simulink model "TST_EnumTypes"  (Simulink 7.4)
settings: Solver=FixedStepDiscrete  StartTime=0.0  StopTime=10.0  FixedStep=0.02  RelTol=1e-3
undefined symbols (not defined in the file): DIL_VmmGsFcsCommandsMessage_LatApModeCmd, DIL_VmmGsFcsCommandsMessage_LongApModeCmd
settings Model: Creator=kharthforeign  LastModifiedBy=kharthforeign  BufferReuse=off
settings DataIOCC: SaveOutput=off  SignalLogging=off  SaveTime=off
settings OptimizationCC: BlockReduction=off  ConditionallyExecuteInputs=off  OptimizeBlockIOStorage=off  BufferReuse=off  ExpressionFolding=off  LocalBlockOutputs=off  InitFltsAndDblsToZero=on

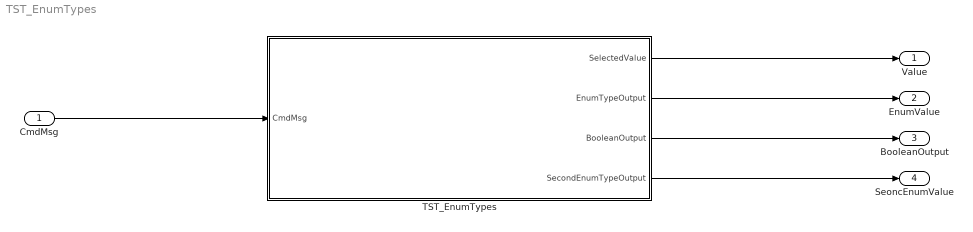
== system TST_EnumTypes ==
  CmdMsg : Inport  UseBusObject=on  OutDataType=fixdt(1, 16)  OutScaling=2^0  BusOutputAsStruct=on
      settings: BusObject=DIL_VmmGsFcsCommandsMessage_Data
  TST_EnumTypes : Subsystem  TreatAsAtomicUnit=on
  Value : Outport  PortDimensions=1  DataType=double  OutDataType=fixdt(1, 16)  OutScaling=2^0  OutDataTypeStr=double
  EnumValue : Outport  Port=2  PortDimensions=1  DataType=Specify via dialog  OutDataType=Enum: DIL_VmmGsFcsCommandsMessage_LongApModeCmd  OutDataTypeStr=Enum: DIL_VmmGsFcsCommandsMessage_LongApModeCmd
  BooleanOutput : Outport  Port=3  PortDimensions=1  DataType=boolean  OutDataType=fixdt(1, 16)  OutScaling=2^0  OutDataTypeStr=boolean
  SeoncEnumValue : Outport  Port=4  PortDimensions=1  DataType=Specify via dialog  OutDataType=Enum: DIL_VmmGsFcsCommandsMessage_LongApModeCmd  OutDataTypeStr=Enum: DIL_VmmGsFcsCommandsMessage_LongApModeCmd
  wires:
  CmdMsg/1 -> TST_EnumTypes/1(CmdMsg)
  TST_EnumTypes/1(SelectedValue) -> Value/1
  TST_EnumTypes/2(EnumTypeOutput) -> EnumValue/1
  TST_EnumTypes/3(BooleanOutput) -> BooleanOutput/1
  TST_EnumTypes/4(SecondEnumTypeOutput) -> SeoncEnumValue/1

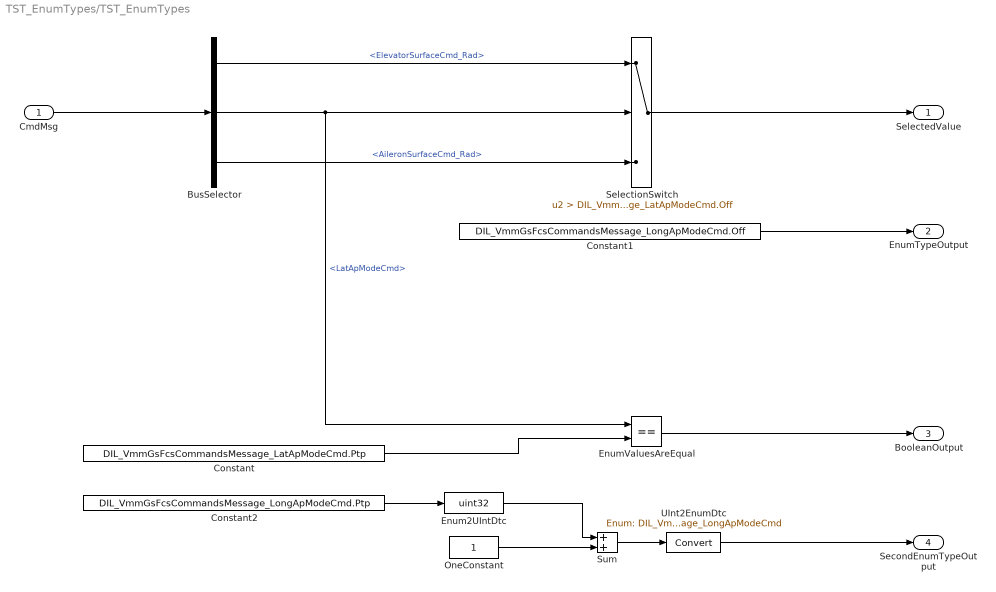
== system TST_EnumTypes/TST_EnumTypes ==
  CmdMsg : Inport  UseBusObject=on  OutDataType=fixdt(1, 16)  OutScaling=2^0
      settings: BusObject=DIL_VmmGsFcsCommandsMessage_Data
  BusSelector : BusSelector  OutputSignals=ElevatorSurfaceCmd_Rad,LatApModeCmd,AileronSurfaceCmd_Rad
  Constant : Constant  Value=DIL_VmmGsFcsCommandsMessage_LatApModeCmd.Ptp  OutDataTypeMode=Specify via dialog  OutDataType=Enum: DIL_VmmGsFcsCommandsMessage_LatApModeCmd  ConRadixGroup=Best Precision: Vector-wise  OutDataTypeStr=Enum: DIL_VmmGsFcsCommandsMessage_LatApModeCmd
  Constant1 : Constant  Value=DIL_VmmGsFcsCommandsMessage_LongApModeCmd.Off  OutDataType=Enum: DIL_VmmGsFcsCommandsMessage_LatApModeCmd  ConRadixGroup=Best Precision: Vector-wise
  Constant2 : Constant  Value=DIL_VmmGsFcsCommandsMessage_LongApModeCmd.Ptp  OutDataType=Enum: DIL_VmmGsFcsCommandsMessage_LatApModeCmd  ConRadixGroup=Best Precision: Vector-wise
  Enum2UIntDtc : DataTypeConversion  OutDataTypeMode=uint32  OutDataType=fixdt(1, 16)  OutScaling=2^0  OutDataTypeStr=uint32
  EnumValuesAreEqual : RelationalOperator  Operator===  LogicOutDataTypeMode=boolean  LogicDataType=fixdt(0, 8)  OutDataTypeStr=boolean
  OneConstant : Constant  OutDataTypeMode=uint32  OutDataType=fixdt(1, 16)  OutScaling=2^0  OutDataTypeStr=uint32
  SelectionSwitch : Switch  Criteria=u2 > Threshold  Threshold=DIL_VmmGsFcsCommandsMessage_LatApModeCmd.Off  OutDataType=fixdt(1, 16)  OutScaling=2^0
  Sum : Sum  OutDataType=fixdt(1, 16)  OutScaling=2^0
  UInt2EnumDtc : DataTypeConversion  OutDataTypeMode=Specify via dialog  OutDataType=Enum: DIL_VmmGsFcsCommandsMessage_LongApModeCmd  OutDataTypeStr=Enum: DIL_VmmGsFcsCommandsMessage_LongApModeCmd
  SelectedValue : Outport  PortDimensions=1  DataType=double  OutDataType=fixdt(1, 16)  OutScaling=2^0  OutDataTypeStr=double
  EnumTypeOutput : Outport  Port=2  PortDimensions=1  DataType=Specify via dialog  OutDataType=Enum: DIL_VmmGsFcsCommandsMessage_LongApModeCmd  OutDataTypeStr=Enum: DIL_VmmGsFcsCommandsMessage_LongApModeCmd
  BooleanOutput : Outport  Port=3  PortDimensions=1  DataType=boolean  OutDataType=fixdt(1, 16)  OutScaling=2^0  OutDataTypeStr=boolean
  SecondEnumTypeOutput : Outport  Port=4  PortDimensions=1  DataType=Specify via dialog  OutDataType=Enum: DIL_VmmGsFcsCommandsMessage_LongApModeCmd  OutDataTypeStr=Enum: DIL_VmmGsFcsCommandsMessage_LongApModeCmd
  wires:
  CmdMsg/1 -> BusSelector/1
  SelectionSwitch/1 -> SelectedValue/1
  BusSelector/1 -> SelectionSwitch/1  "<ElevatorSurfaceCmd_Rad>"
  BusSelector/3 -> SelectionSwitch/3  "<AileronSurfaceCmd_Rad>"
  BusSelector/2 -> SelectionSwitch/2, EnumValuesAreEqual/1  "<LatApModeCmd>"
  Constant1/1 -> EnumTypeOutput/1
  EnumValuesAreEqual/1 -> BooleanOutput/1
  Constant/1 -> EnumValuesAreEqual/2
  Constant2/1 -> Enum2UIntDtc/1
  Enum2UIntDtc/1 -> Sum/1
  Sum/1 -> UInt2EnumDtc/1
  UInt2EnumDtc/1 -> SecondEnumTypeOutput/1
  OneConstant/1 -> Sum/2
